simulink model "qless_forgetting_factor_16x16_nofifo"  (R2021a)
settings: Solver=FixedStepDiscrete  StartTime=0.0  StopTime=stoptime*inf  RelTol=1e-3
InitFcn:
  | qless_init_16chan_fi
undefined symbols (not defined in the file): fc, numArrayElements, physconst, srcAngles, Ts
libraries: hdlsllib x137, commfilt2 x4, commrfcorlib x3, commsync2 x3, commrflib2 x2, commrandsrc3 x2, simulink x2, phasedtxrxlib x2, commdigbbndcpm2 x1, embreciprocals x1, commdigbbndpm3 x1
(part 3 of 22)

== system qless_forgetting_factor_16x16_nofifo/MVDR_QLess_HDL/Complex Partial-Systolic Matrix Solve Using Q-less QR Decomposition with Forgetting Factor Manually Tiled n=16/Complex Partial-Systolic Q-less QR with Forgetting Factor/Complex Partial-Systolic Q-less QR with Forgetting Factor Manually tiled/Complex Partial-Systolic Q-less QR Decomposition with Forgetting Factor Section Constant pivot10 ==
  "A(i, :)^T" : Inport
  validIn : Inport  Port=2
  restart : Inport  Port=3
  Complex Partial-Systolic Q-less QR Row Rotations : Subsystem  mask(QR Complex Row Rotations){n=n, pivot=pivot}
      mask prompts: n "fixed:emblib:ColumnsInA"
      mask help: fixed:emblib:ComplexRowRotationsFullDescription
      mask DialogControl n Prompt: Number of columns in matrix A
  Data Type Conversion{,2..6} (6 alike) : DataTypeConversion  OutDataTypeStr=boolean
  Forgetting Factor : Gain  Gain=forgettingFactor  OutDataTypeStr=Inherit: Same as input
  Partial-Systolic Q-less QR with Forgetting Factor Memory Controller : Subsystem  TreatAsAtomicUnit=on  mask(Burst Q-less QR QR Memory Controller){n=n}
      mask prompts: n "fixed:emblib:ColumnsInA"
      mask help: fixed:emblib:MemoryControllerDescription
      mask DialogControl n Prompt: Number of columns in matrix A
  Same Datatype : Subsystem  TreatAsAtomicUnit=on
  Terminator : Terminator
  "R(i, :)^T" : Outport  VectorParamsAs1DForOutWhenUnconnected=off
  validR : Outport  Port=2  VectorParamsAs1DForOutWhenUnconnected=off
  yOut : Outport  Port=3  VectorParamsAs1DForOutWhenUnconnected=off
  validY : Outport  Port=4  VectorParamsAs1DForOutWhenUnconnected=off
  ready : Outport  Port=5  VectorParamsAs1DForOutWhenUnconnected=off
  wires:
  "A(i, :)^T"/1 -> Same Datatype/2(Reference), Partial-Systolic Q-less QR with Forgetting Factor Memory Controller/2(aIn)
  restart/1 -> Data Type Conversion2/1
  Complex Partial-Systolic Q-less QR Row Rotations/3(validOut) -> Data Type Conversion3/1
  Partial-Systolic Q-less QR with Forgetting Factor Memory Controller/4(validOut) -> Data Type Conversion5/1
  validIn/1 -> Data Type Conversion/1
  Partial-Systolic Q-less QR with Forgetting Factor Memory Controller/2(yOut) -> Complex Partial-Systolic Q-less QR Row Rotations/2(y)
  Same Datatype/1(DataOut) -> Partial-Systolic Q-less QR with Forgetting Factor Memory Controller/1(xIn)
  Partial-Systolic Q-less QR with Forgetting Factor Memory Controller/5(ready) -> Data Type Conversion6/1
  Complex Partial-Systolic Q-less QR Row Rotations/2(yOut) -> yOut/1
  Complex Partial-Systolic Q-less QR Row Rotations/4(ready) -> Terminator/1
  Partial-Systolic Q-less QR with Forgetting Factor Memory Controller/3(process) -> Data Type Conversion4/1
  Complex Partial-Systolic Q-less QR Row Rotations/1(xOut) -> Forgetting Factor/1
  Partial-Systolic Q-less QR with Forgetting Factor Memory Controller/1(xOut) -> Complex Partial-Systolic Q-less QR Row Rotations/1(x), "R(i, :)^T"/1
  Forgetting Factor/1 -> Same Datatype/1(Data)
  Data Type Conversion/1 -> Partial-Systolic Q-less QR with Forgetting Factor Memory Controller/3(validIn)
  Data Type Conversion2/1 -> Complex Partial-Systolic Q-less QR Row Rotations/4(restart), Partial-Systolic Q-less QR with Forgetting Factor Memory Controller/5(restart)
  Data Type Conversion3/1 -> Partial-Systolic Q-less QR with Forgetting Factor Memory Controller/4(validElim), validY/1
  Data Type Conversion5/1 -> validR/1
  Data Type Conversion6/1 -> ready/1
  Data Type Conversion4/1 -> Complex Partial-Systolic Q-less QR Row Rotations/3(validIn)

== system qless_forgetting_factor_16x16_nofifo/MVDR_QLess_HDL/Complex Partial-Systolic Matrix Solve Using Q-less QR Decomposition with Forgetting Factor Manually Tiled n=16/Complex Partial-Systolic Q-less QR with Forgetting Factor/Complex Partial-Systolic Q-less QR with Forgetting Factor Manually tiled/Complex Partial-Systolic Q-less QR Decomposition with Forgetting Factor Section Constant pivot11 ==
  "A(i, :)^T" : Inport
  validIn : Inport  Port=2
  restart : Inport  Port=3
  Complex Partial-Systolic Q-less QR Row Rotations : Subsystem  mask(QR Complex Row Rotations){n=n, pivot=pivot}
      mask prompts: n "fixed:emblib:ColumnsInA"
      mask help: fixed:emblib:ComplexRowRotationsFullDescription
      mask DialogControl n Prompt: Number of columns in matrix A
  Data Type Conversion{,2..6} (6 alike) : DataTypeConversion  OutDataTypeStr=boolean
  Forgetting Factor : Gain  Gain=forgettingFactor  OutDataTypeStr=Inherit: Same as input
  Partial-Systolic Q-less QR with Forgetting Factor Memory Controller : Subsystem  TreatAsAtomicUnit=on  mask(Burst Q-less QR QR Memory Controller){n=n}
      mask prompts: n "fixed:emblib:ColumnsInA"
      mask help: fixed:emblib:MemoryControllerDescription
      mask DialogControl n Prompt: Number of columns in matrix A
  Same Datatype : Subsystem  TreatAsAtomicUnit=on
  Terminator : Terminator
  "R(i, :)^T" : Outport  VectorParamsAs1DForOutWhenUnconnected=off
  validR : Outport  Port=2  VectorParamsAs1DForOutWhenUnconnected=off
  yOut : Outport  Port=3  VectorParamsAs1DForOutWhenUnconnected=off
  validY : Outport  Port=4  VectorParamsAs1DForOutWhenUnconnected=off
  ready : Outport  Port=5  VectorParamsAs1DForOutWhenUnconnected=off
  wires:
  "A(i, :)^T"/1 -> Same Datatype/2(Reference), Partial-Systolic Q-less QR with Forgetting Factor Memory Controller/2(aIn)
  restart/1 -> Data Type Conversion2/1
  Complex Partial-Systolic Q-less QR Row Rotations/3(validOut) -> Data Type Conversion3/1
  Partial-Systolic Q-less QR with Forgetting Factor Memory Controller/4(validOut) -> Data Type Conversion5/1
  validIn/1 -> Data Type Conversion/1
  Partial-Systolic Q-less QR with Forgetting Factor Memory Controller/2(yOut) -> Complex Partial-Systolic Q-less QR Row Rotations/2(y)
  Same Datatype/1(DataOut) -> Partial-Systolic Q-less QR with Forgetting Factor Memory Controller/1(xIn)
  Partial-Systolic Q-less QR with Forgetting Factor Memory Controller/5(ready) -> Data Type Conversion6/1
  Complex Partial-Systolic Q-less QR Row Rotations/2(yOut) -> yOut/1
  Complex Partial-Systolic Q-less QR Row Rotations/4(ready) -> Terminator/1
  Partial-Systolic Q-less QR with Forgetting Factor Memory Controller/3(process) -> Data Type Conversion4/1
  Complex Partial-Systolic Q-less QR Row Rotations/1(xOut) -> Forgetting Factor/1
  Partial-Systolic Q-less QR with Forgetting Factor Memory Controller/1(xOut) -> Complex Partial-Systolic Q-less QR Row Rotations/1(x), "R(i, :)^T"/1
  Forgetting Factor/1 -> Same Datatype/1(Data)
  Data Type Conversion/1 -> Partial-Systolic Q-less QR with Forgetting Factor Memory Controller/3(validIn)
  Data Type Conversion2/1 -> Complex Partial-Systolic Q-less QR Row Rotations/4(restart), Partial-Systolic Q-less QR with Forgetting Factor Memory Controller/5(restart)
  Data Type Conversion3/1 -> Partial-Systolic Q-less QR with Forgetting Factor Memory Controller/4(validElim), validY/1
  Data Type Conversion5/1 -> validR/1
  Data Type Conversion6/1 -> ready/1
  Data Type Conversion4/1 -> Complex Partial-Systolic Q-less QR Row Rotations/3(validIn)

== system qless_forgetting_factor_16x16_nofifo/MVDR_QLess_HDL/Complex Partial-Systolic Matrix Solve Using Q-less QR Decomposition with Forgetting Factor Manually Tiled n=16/Complex Partial-Systolic Q-less QR with Forgetting Factor/Complex Partial-Systolic Q-less QR with Forgetting Factor Manually tiled/Complex Partial-Systolic Q-less QR Decomposition with Forgetting Factor Section Constant pivot12 ==
  "A(i, :)^T" : Inport
  validIn : Inport  Port=2
  restart : Inport  Port=3
  Complex Partial-Systolic Q-less QR Row Rotations : Subsystem  mask(QR Complex Row Rotations){n=n, pivot=pivot}
      mask prompts: n "fixed:emblib:ColumnsInA"
      mask help: fixed:emblib:ComplexRowRotationsFullDescription
      mask DialogControl n Prompt: Number of columns in matrix A
  Data Type Conversion{,2..6} (6 alike) : DataTypeConversion  OutDataTypeStr=boolean
  Forgetting Factor : Gain  Gain=forgettingFactor  OutDataTypeStr=Inherit: Same as input
  Partial-Systolic Q-less QR with Forgetting Factor Memory Controller : Subsystem  TreatAsAtomicUnit=on  mask(Burst Q-less QR QR Memory Controller){n=n}
      mask prompts: n "fixed:emblib:ColumnsInA"
      mask help: fixed:emblib:MemoryControllerDescription
      mask DialogControl n Prompt: Number of columns in matrix A
  Same Datatype : Subsystem  TreatAsAtomicUnit=on
  Terminator : Terminator
  "R(i, :)^T" : Outport  VectorParamsAs1DForOutWhenUnconnected=off
  validR : Outport  Port=2  VectorParamsAs1DForOutWhenUnconnected=off
  yOut : Outport  Port=3  VectorParamsAs1DForOutWhenUnconnected=off
  validY : Outport  Port=4  VectorParamsAs1DForOutWhenUnconnected=off
  ready : Outport  Port=5  VectorParamsAs1DForOutWhenUnconnected=off
  wires:
  "A(i, :)^T"/1 -> Same Datatype/2(Reference), Partial-Systolic Q-less QR with Forgetting Factor Memory Controller/2(aIn)
  restart/1 -> Data Type Conversion2/1
  Complex Partial-Systolic Q-less QR Row Rotations/3(validOut) -> Data Type Conversion3/1
  Partial-Systolic Q-less QR with Forgetting Factor Memory Controller/4(validOut) -> Data Type Conversion5/1
  validIn/1 -> Data Type Conversion/1
  Partial-Systolic Q-less QR with Forgetting Factor Memory Controller/2(yOut) -> Complex Partial-Systolic Q-less QR Row Rotations/2(y)
  Same Datatype/1(DataOut) -> Partial-Systolic Q-less QR with Forgetting Factor Memory Controller/1(xIn)
  Partial-Systolic Q-less QR with Forgetting Factor Memory Controller/5(ready) -> Data Type Conversion6/1
  Complex Partial-Systolic Q-less QR Row Rotations/2(yOut) -> yOut/1
  Complex Partial-Systolic Q-less QR Row Rotations/4(ready) -> Terminator/1
  Partial-Systolic Q-less QR with Forgetting Factor Memory Controller/3(process) -> Data Type Conversion4/1
  Complex Partial-Systolic Q-less QR Row Rotations/1(xOut) -> Forgetting Factor/1
  Partial-Systolic Q-less QR with Forgetting Factor Memory Controller/1(xOut) -> Complex Partial-Systolic Q-less QR Row Rotations/1(x), "R(i, :)^T"/1
  Forgetting Factor/1 -> Same Datatype/1(Data)
  Data Type Conversion/1 -> Partial-Systolic Q-less QR with Forgetting Factor Memory Controller/3(validIn)
  Data Type Conversion2/1 -> Complex Partial-Systolic Q-less QR Row Rotations/4(restart), Partial-Systolic Q-less QR with Forgetting Factor Memory Controller/5(restart)
  Data Type Conversion3/1 -> Partial-Systolic Q-less QR with Forgetting Factor Memory Controller/4(validElim), validY/1
  Data Type Conversion5/1 -> validR/1
  Data Type Conversion6/1 -> ready/1
  Data Type Conversion4/1 -> Complex Partial-Systolic Q-less QR Row Rotations/3(validIn)

== system qless_forgetting_factor_16x16_nofifo/MVDR_QLess_HDL/Complex Partial-Systolic Matrix Solve Using Q-less QR Decomposition with Forgetting Factor Manually Tiled n=16/Complex Partial-Systolic Q-less QR with Forgetting Factor/Complex Partial-Systolic Q-less QR with Forgetting Factor Manually tiled/Complex Partial-Systolic Q-less QR Decomposition with Forgetting Factor Section Constant pivot13 ==
  "A(i, :)^T" : Inport
  validIn : Inport  Port=2
  restart : Inport  Port=3
  Complex Partial-Systolic Q-less QR Row Rotations : Subsystem  mask(QR Complex Row Rotations){n=n, pivot=pivot}
      mask prompts: n "fixed:emblib:ColumnsInA"
      mask help: fixed:emblib:ComplexRowRotationsFullDescription
      mask DialogControl n Prompt: Number of columns in matrix A
  Data Type Conversion{,2..6} (6 alike) : DataTypeConversion  OutDataTypeStr=boolean
  Forgetting Factor : Gain  Gain=forgettingFactor  OutDataTypeStr=Inherit: Same as input
  Partial-Systolic Q-less QR with Forgetting Factor Memory Controller : Subsystem  TreatAsAtomicUnit=on  mask(Burst Q-less QR QR Memory Controller){n=n}
      mask prompts: n "fixed:emblib:ColumnsInA"
      mask help: fixed:emblib:MemoryControllerDescription
      mask DialogControl n Prompt: Number of columns in matrix A
  Same Datatype : Subsystem  TreatAsAtomicUnit=on
  Terminator : Terminator
  "R(i, :)^T" : Outport  VectorParamsAs1DForOutWhenUnconnected=off
  validR : Outport  Port=2  VectorParamsAs1DForOutWhenUnconnected=off
  yOut : Outport  Port=3  VectorParamsAs1DForOutWhenUnconnected=off
  validY : Outport  Port=4  VectorParamsAs1DForOutWhenUnconnected=off
  ready : Outport  Port=5  VectorParamsAs1DForOutWhenUnconnected=off
  wires:
  "A(i, :)^T"/1 -> Same Datatype/2(Reference), Partial-Systolic Q-less QR with Forgetting Factor Memory Controller/2(aIn)
  restart/1 -> Data Type Conversion2/1
  Complex Partial-Systolic Q-less QR Row Rotations/3(validOut) -> Data Type Conversion3/1
  Partial-Systolic Q-less QR with Forgetting Factor Memory Controller/4(validOut) -> Data Type Conversion5/1
  validIn/1 -> Data Type Conversion/1
  Partial-Systolic Q-less QR with Forgetting Factor Memory Controller/2(yOut) -> Complex Partial-Systolic Q-less QR Row Rotations/2(y)
  Same Datatype/1(DataOut) -> Partial-Systolic Q-less QR with Forgetting Factor Memory Controller/1(xIn)
  Partial-Systolic Q-less QR with Forgetting Factor Memory Controller/5(ready) -> Data Type Conversion6/1
  Complex Partial-Systolic Q-less QR Row Rotations/2(yOut) -> yOut/1
  Complex Partial-Systolic Q-less QR Row Rotations/4(ready) -> Terminator/1
  Partial-Systolic Q-less QR with Forgetting Factor Memory Controller/3(process) -> Data Type Conversion4/1
  Complex Partial-Systolic Q-less QR Row Rotations/1(xOut) -> Forgetting Factor/1
  Partial-Systolic Q-less QR with Forgetting Factor Memory Controller/1(xOut) -> Complex Partial-Systolic Q-less QR Row Rotations/1(x), "R(i, :)^T"/1
  Forgetting Factor/1 -> Same Datatype/1(Data)
  Data Type Conversion/1 -> Partial-Systolic Q-less QR with Forgetting Factor Memory Controller/3(validIn)
  Data Type Conversion2/1 -> Complex Partial-Systolic Q-less QR Row Rotations/4(restart), Partial-Systolic Q-less QR with Forgetting Factor Memory Controller/5(restart)
  Data Type Conversion3/1 -> Partial-Systolic Q-less QR with Forgetting Factor Memory Controller/4(validElim), validY/1
  Data Type Conversion5/1 -> validR/1
  Data Type Conversion6/1 -> ready/1
  Data Type Conversion4/1 -> Complex Partial-Systolic Q-less QR Row Rotations/3(validIn)

== system qless_forgetting_factor_16x16_nofifo/MVDR_QLess_HDL/Complex Partial-Systolic Matrix Solve Using Q-less QR Decomposition with Forgetting Factor Manually Tiled n=16/Complex Partial-Systolic Q-less QR with Forgetting Factor/Complex Partial-Systolic Q-less QR with Forgetting Factor Manually tiled/Complex Partial-Systolic Q-less QR Decomposition with Forgetting Factor Section Constant pivot14 ==
  "A(i, :)^T" : Inport
  validIn : Inport  Port=2
  restart : Inport  Port=3
  Complex Partial-Systolic Q-less QR Row Rotations : Subsystem  mask(QR Complex Row Rotations){n=n, pivot=pivot}
      mask prompts: n "fixed:emblib:ColumnsInA"
      mask help: fixed:emblib:ComplexRowRotationsFullDescription
      mask DialogControl n Prompt: Number of columns in matrix A
  Data Type Conversion{,2..6} (6 alike) : DataTypeConversion  OutDataTypeStr=boolean
  Forgetting Factor : Gain  Gain=forgettingFactor  OutDataTypeStr=Inherit: Same as input
  Partial-Systolic Q-less QR with Forgetting Factor Memory Controller : Subsystem  TreatAsAtomicUnit=on  mask(Burst Q-less QR QR Memory Controller){n=n}
      mask prompts: n "fixed:emblib:ColumnsInA"
      mask help: fixed:emblib:MemoryControllerDescription
      mask DialogControl n Prompt: Number of columns in matrix A
  Same Datatype : Subsystem  TreatAsAtomicUnit=on
  Terminator : Terminator
  "R(i, :)^T" : Outport  VectorParamsAs1DForOutWhenUnconnected=off
  validR : Outport  Port=2  VectorParamsAs1DForOutWhenUnconnected=off
  yOut : Outport  Port=3  VectorParamsAs1DForOutWhenUnconnected=off
  validY : Outport  Port=4  VectorParamsAs1DForOutWhenUnconnected=off
  ready : Outport  Port=5  VectorParamsAs1DForOutWhenUnconnected=off
  wires:
  "A(i, :)^T"/1 -> Same Datatype/2(Reference), Partial-Systolic Q-less QR with Forgetting Factor Memory Controller/2(aIn)
  restart/1 -> Data Type Conversion2/1
  Complex Partial-Systolic Q-less QR Row Rotations/3(validOut) -> Data Type Conversion3/1
  Partial-Systolic Q-less QR with Forgetting Factor Memory Controller/4(validOut) -> Data Type Conversion5/1
  validIn/1 -> Data Type Conversion/1
  Partial-Systolic Q-less QR with Forgetting Factor Memory Controller/2(yOut) -> Complex Partial-Systolic Q-less QR Row Rotations/2(y)
  Same Datatype/1(DataOut) -> Partial-Systolic Q-less QR with Forgetting Factor Memory Controller/1(xIn)
  Partial-Systolic Q-less QR with Forgetting Factor Memory Controller/5(ready) -> Data Type Conversion6/1
  Complex Partial-Systolic Q-less QR Row Rotations/2(yOut) -> yOut/1
  Complex Partial-Systolic Q-less QR Row Rotations/4(ready) -> Terminator/1
  Partial-Systolic Q-less QR with Forgetting Factor Memory Controller/3(process) -> Data Type Conversion4/1
  Complex Partial-Systolic Q-less QR Row Rotations/1(xOut) -> Forgetting Factor/1
  Partial-Systolic Q-less QR with Forgetting Factor Memory Controller/1(xOut) -> Complex Partial-Systolic Q-less QR Row Rotations/1(x), "R(i, :)^T"/1
  Forgetting Factor/1 -> Same Datatype/1(Data)
  Data Type Conversion/1 -> Partial-Systolic Q-less QR with Forgetting Factor Memory Controller/3(validIn)
  Data Type Conversion2/1 -> Complex Partial-Systolic Q-less QR Row Rotations/4(restart), Partial-Systolic Q-less QR with Forgetting Factor Memory Controller/5(restart)
  Data Type Conversion3/1 -> Partial-Systolic Q-less QR with Forgetting Factor Memory Controller/4(validElim), validY/1
  Data Type Conversion5/1 -> validR/1
  Data Type Conversion6/1 -> ready/1
  Data Type Conversion4/1 -> Complex Partial-Systolic Q-less QR Row Rotations/3(validIn)

== system qless_forgetting_factor_16x16_nofifo/MVDR_QLess_HDL/Complex Partial-Systolic Matrix Solve Using Q-less QR Decomposition with Forgetting Factor Manually Tiled n=16/Complex Partial-Systolic Q-less QR with Forgetting Factor/Complex Partial-Systolic Q-less QR with Forgetting Factor Manually tiled/Complex Partial-Systolic Q-less QR Decomposition with Forgetting Factor Section Constant pivot15 ==
  "A(i, :)^T" : Inport
  validIn : Inport  Port=2
  restart : Inport  Port=3
  Complex Partial-Systolic Q-less QR Row Rotations : Subsystem  mask(QR Complex Row Rotations){n=n, pivot=pivot}
      mask prompts: n "fixed:emblib:ColumnsInA"
      mask help: fixed:emblib:ComplexRowRotationsFullDescription
      mask DialogControl n Prompt: Number of columns in matrix A
  Data Type Conversion{,2..6} (6 alike) : DataTypeConversion  OutDataTypeStr=boolean
  Forgetting Factor : Gain  Gain=forgettingFactor  OutDataTypeStr=Inherit: Same as input
  Partial-Systolic Q-less QR with Forgetting Factor Memory Controller : Subsystem  TreatAsAtomicUnit=on  mask(Burst Q-less QR QR Memory Controller){n=n}
      mask prompts: n "fixed:emblib:ColumnsInA"
      mask help: fixed:emblib:MemoryControllerDescription
      mask DialogControl n Prompt: Number of columns in matrix A
  Same Datatype : Subsystem  TreatAsAtomicUnit=on
  Terminator : Terminator
  "R(i, :)^T" : Outport  VectorParamsAs1DForOutWhenUnconnected=off
  validR : Outport  Port=2  VectorParamsAs1DForOutWhenUnconnected=off
  yOut : Outport  Port=3  VectorParamsAs1DForOutWhenUnconnected=off
  validY : Outport  Port=4  VectorParamsAs1DForOutWhenUnconnected=off
  ready : Outport  Port=5  VectorParamsAs1DForOutWhenUnconnected=off
  wires:
  "A(i, :)^T"/1 -> Same Datatype/2(Reference), Partial-Systolic Q-less QR with Forgetting Factor Memory Controller/2(aIn)
  restart/1 -> Data Type Conversion2/1
  Complex Partial-Systolic Q-less QR Row Rotations/3(validOut) -> Data Type Conversion3/1
  Partial-Systolic Q-less QR with Forgetting Factor Memory Controller/4(validOut) -> Data Type Conversion5/1
  validIn/1 -> Data Type Conversion/1
  Partial-Systolic Q-less QR with Forgetting Factor Memory Controller/2(yOut) -> Complex Partial-Systolic Q-less QR Row Rotations/2(y)
  Same Datatype/1(DataOut) -> Partial-Systolic Q-less QR with Forgetting Factor Memory Controller/1(xIn)
  Partial-Systolic Q-less QR with Forgetting Factor Memory Controller/5(ready) -> Data Type Conversion6/1
  Complex Partial-Systolic Q-less QR Row Rotations/2(yOut) -> yOut/1
  Complex Partial-Systolic Q-less QR Row Rotations/4(ready) -> Terminator/1
  Partial-Systolic Q-less QR with Forgetting Factor Memory Controller/3(process) -> Data Type Conversion4/1
  Complex Partial-Systolic Q-less QR Row Rotations/1(xOut) -> Forgetting Factor/1
  Partial-Systolic Q-less QR with Forgetting Factor Memory Controller/1(xOut) -> Complex Partial-Systolic Q-less QR Row Rotations/1(x), "R(i, :)^T"/1
  Forgetting Factor/1 -> Same Datatype/1(Data)
  Data Type Conversion/1 -> Partial-Systolic Q-less QR with Forgetting Factor Memory Controller/3(validIn)
  Data Type Conversion2/1 -> Complex Partial-Systolic Q-less QR Row Rotations/4(restart), Partial-Systolic Q-less QR with Forgetting Factor Memory Controller/5(restart)
  Data Type Conversion3/1 -> Partial-Systolic Q-less QR with Forgetting Factor Memory Controller/4(validElim), validY/1
  Data Type Conversion5/1 -> validR/1
  Data Type Conversion6/1 -> ready/1
  Data Type Conversion4/1 -> Complex Partial-Systolic Q-less QR Row Rotations/3(validIn)

== system qless_forgetting_factor_16x16_nofifo/MVDR_QLess_HDL/Complex Partial-Systolic Matrix Solve Using Q-less QR Decomposition with Forgetting Factor Manually Tiled n=16/Complex Partial-Systolic Q-less QR with Forgetting Factor/Complex Partial-Systolic Q-less QR with Forgetting Factor Manually tiled/Complex Partial-Systolic Q-less QR Decomposition with Forgetting Factor Section Constant pivot16 ==
  "A(i, :)^T" : Inport
  validIn : Inport  Port=2
  restart : Inport  Port=3
  Complex Partial-Systolic Q-less QR Row Rotations : Subsystem  mask(QR Complex Row Rotations){n=n, pivot=pivot}
      mask prompts: n "fixed:emblib:ColumnsInA"
      mask help: fixed:emblib:ComplexRowRotationsFullDescription
      mask DialogControl n Prompt: Number of columns in matrix A
  Data Type Conversion{,2..6} (6 alike) : DataTypeConversion  OutDataTypeStr=boolean
  Forgetting Factor : Gain  Gain=forgettingFactor  OutDataTypeStr=Inherit: Same as input
  Partial-Systolic Q-less QR with Forgetting Factor Memory Controller : Subsystem  TreatAsAtomicUnit=on  mask(Burst Q-less QR QR Memory Controller){n=n}
      mask prompts: n "fixed:emblib:ColumnsInA"
      mask help: fixed:emblib:MemoryControllerDescription
      mask DialogControl n Prompt: Number of columns in matrix A
  Same Datatype : Subsystem  TreatAsAtomicUnit=on
  Terminator : Terminator
  "R(i, :)^T" : Outport  VectorParamsAs1DForOutWhenUnconnected=off
  validR : Outport  Port=2  VectorParamsAs1DForOutWhenUnconnected=off
  yOut : Outport  Port=3  VectorParamsAs1DForOutWhenUnconnected=off
  validY : Outport  Port=4  VectorParamsAs1DForOutWhenUnconnected=off
  ready : Outport  Port=5  VectorParamsAs1DForOutWhenUnconnected=off
  wires:
  "A(i, :)^T"/1 -> Same Datatype/2(Reference), Partial-Systolic Q-less QR with Forgetting Factor Memory Controller/2(aIn)
  restart/1 -> Data Type Conversion2/1
  Complex Partial-Systolic Q-less QR Row Rotations/3(validOut) -> Data Type Conversion3/1
  Partial-Systolic Q-less QR with Forgetting Factor Memory Controller/4(validOut) -> Data Type Conversion5/1
  validIn/1 -> Data Type Conversion/1
  Partial-Systolic Q-less QR with Forgetting Factor Memory Controller/2(yOut) -> Complex Partial-Systolic Q-less QR Row Rotations/2(y)
  Same Datatype/1(DataOut) -> Partial-Systolic Q-less QR with Forgetting Factor Memory Controller/1(xIn)
  Partial-Systolic Q-less QR with Forgetting Factor Memory Controller/5(ready) -> Data Type Conversion6/1
  Complex Partial-Systolic Q-less QR Row Rotations/2(yOut) -> yOut/1
  Complex Partial-Systolic Q-less QR Row Rotations/4(ready) -> Terminator/1
  Partial-Systolic Q-less QR with Forgetting Factor Memory Controller/3(process) -> Data Type Conversion4/1
  Complex Partial-Systolic Q-less QR Row Rotations/1(xOut) -> Forgetting Factor/1
  Partial-Systolic Q-less QR with Forgetting Factor Memory Controller/1(xOut) -> Complex Partial-Systolic Q-less QR Row Rotations/1(x), "R(i, :)^T"/1
  Forgetting Factor/1 -> Same Datatype/1(Data)
  Data Type Conversion/1 -> Partial-Systolic Q-less QR with Forgetting Factor Memory Controller/3(validIn)
  Data Type Conversion2/1 -> Complex Partial-Systolic Q-less QR Row Rotations/4(restart), Partial-Systolic Q-less QR with Forgetting Factor Memory Controller/5(restart)
  Data Type Conversion3/1 -> Partial-Systolic Q-less QR with Forgetting Factor Memory Controller/4(validElim), validY/1
  Data Type Conversion5/1 -> validR/1
  Data Type Conversion6/1 -> ready/1
  Data Type Conversion4/1 -> Complex Partial-Systolic Q-less QR Row Rotations/3(validIn)

== system qless_forgetting_factor_16x16_nofifo/MVDR_QLess_HDL/Complex Partial-Systolic Matrix Solve Using Q-less QR Decomposition with Forgetting Factor Manually Tiled n=16/Complex Partial-Systolic Q-less QR with Forgetting Factor/Complex Partial-Systolic Q-less QR with Forgetting Factor Manually tiled/Complex Partial-Systolic Q-less QR Decomposition with Forgetting Factor Section Constant pivot2 ==
  "A(i, :)^T" : Inport
  validIn : Inport  Port=2
  restart : Inport  Port=3
  Complex Partial-Systolic Q-less QR Row Rotations : Subsystem  mask(QR Complex Row Rotations){n=n, pivot=pivot}
      mask prompts: n "fixed:emblib:ColumnsInA"
      mask help: fixed:emblib:ComplexRowRotationsFullDescription
      mask DialogControl n Prompt: Number of columns in matrix A
  Data Type Conversion{,2..6} (6 alike) : DataTypeConversion  OutDataTypeStr=boolean
  Forgetting Factor : Gain  Gain=forgettingFactor  OutDataTypeStr=Inherit: Same as input
  Partial-Systolic Q-less QR with Forgetting Factor Memory Controller : Subsystem  TreatAsAtomicUnit=on  mask(Burst Q-less QR QR Memory Controller){n=n}
      mask prompts: n "fixed:emblib:ColumnsInA"
      mask help: fixed:emblib:MemoryControllerDescription
      mask DialogControl n Prompt: Number of columns in matrix A
  Same Datatype : Subsystem  TreatAsAtomicUnit=on
  Terminator : Terminator
  "R(i, :)^T" : Outport  VectorParamsAs1DForOutWhenUnconnected=off
  validR : Outport  Port=2  VectorParamsAs1DForOutWhenUnconnected=off
  yOut : Outport  Port=3  VectorParamsAs1DForOutWhenUnconnected=off
  validY : Outport  Port=4  VectorParamsAs1DForOutWhenUnconnected=off
  ready : Outport  Port=5  VectorParamsAs1DForOutWhenUnconnected=off
  wires:
  "A(i, :)^T"/1 -> Same Datatype/2(Reference), Partial-Systolic Q-less QR with Forgetting Factor Memory Controller/2(aIn)
  restart/1 -> Data Type Conversion2/1
  Complex Partial-Systolic Q-less QR Row Rotations/3(validOut) -> Data Type Conversion3/1
  Partial-Systolic Q-less QR with Forgetting Factor Memory Controller/4(validOut) -> Data Type Conversion5/1
  validIn/1 -> Data Type Conversion/1
  Partial-Systolic Q-less QR with Forgetting Factor Memory Controller/2(yOut) -> Complex Partial-Systolic Q-less QR Row Rotations/2(y)
  Same Datatype/1(DataOut) -> Partial-Systolic Q-less QR with Forgetting Factor Memory Controller/1(xIn)
  Partial-Systolic Q-less QR with Forgetting Factor Memory Controller/5(ready) -> Data Type Conversion6/1
  Complex Partial-Systolic Q-less QR Row Rotations/2(yOut) -> yOut/1
  Complex Partial-Systolic Q-less QR Row Rotations/4(ready) -> Terminator/1
  Partial-Systolic Q-less QR with Forgetting Factor Memory Controller/3(process) -> Data Type Conversion4/1
  Complex Partial-Systolic Q-less QR Row Rotations/1(xOut) -> Forgetting Factor/1
  Partial-Systolic Q-less QR with Forgetting Factor Memory Controller/1(xOut) -> Complex Partial-Systolic Q-less QR Row Rotations/1(x), "R(i, :)^T"/1
  Forgetting Factor/1 -> Same Datatype/1(Data)
  Data Type Conversion/1 -> Partial-Systolic Q-less QR with Forgetting Factor Memory Controller/3(validIn)
  Data Type Conversion2/1 -> Complex Partial-Systolic Q-less QR Row Rotations/4(restart), Partial-Systolic Q-less QR with Forgetting Factor Memory Controller/5(restart)
  Data Type Conversion3/1 -> Partial-Systolic Q-less QR with Forgetting Factor Memory Controller/4(validElim), validY/1
  Data Type Conversion5/1 -> validR/1
  Data Type Conversion6/1 -> ready/1
  Data Type Conversion4/1 -> Complex Partial-Systolic Q-less QR Row Rotations/3(validIn)

== system qless_forgetting_factor_16x16_nofifo/MVDR_QLess_HDL/Complex Partial-Systolic Matrix Solve Using Q-less QR Decomposition with Forgetting Factor Manually Tiled n=16/Complex Partial-Systolic Q-less QR with Forgetting Factor/Complex Partial-Systolic Q-less QR with Forgetting Factor Manually tiled/Complex Partial-Systolic Q-less QR Decomposition with Forgetting Factor Section Constant pivot3 ==
  "A(i, :)^T" : Inport
  validIn : Inport  Port=2
  restart : Inport  Port=3
  Complex Partial-Systolic Q-less QR Row Rotations : Subsystem  mask(QR Complex Row Rotations){n=n, pivot=pivot}
      mask prompts: n "fixed:emblib:ColumnsInA"
      mask help: fixed:emblib:ComplexRowRotationsFullDescription
      mask DialogControl n Prompt: Number of columns in matrix A
  Data Type Conversion{,2..6} (6 alike) : DataTypeConversion  OutDataTypeStr=boolean
  Forgetting Factor : Gain  Gain=forgettingFactor  OutDataTypeStr=Inherit: Same as input
  Partial-Systolic Q-less QR with Forgetting Factor Memory Controller : Subsystem  TreatAsAtomicUnit=on  mask(Burst Q-less QR QR Memory Controller){n=n}
      mask prompts: n "fixed:emblib:ColumnsInA"
      mask help: fixed:emblib:MemoryControllerDescription
      mask DialogControl n Prompt: Number of columns in matrix A
  Same Datatype : Subsystem  TreatAsAtomicUnit=on
  Terminator : Terminator
  "R(i, :)^T" : Outport  VectorParamsAs1DForOutWhenUnconnected=off
  validR : Outport  Port=2  VectorParamsAs1DForOutWhenUnconnected=off
  yOut : Outport  Port=3  VectorParamsAs1DForOutWhenUnconnected=off
  validY : Outport  Port=4  VectorParamsAs1DForOutWhenUnconnected=off
  ready : Outport  Port=5  VectorParamsAs1DForOutWhenUnconnected=off
  wires:
  "A(i, :)^T"/1 -> Same Datatype/2(Reference), Partial-Systolic Q-less QR with Forgetting Factor Memory Controller/2(aIn)
  restart/1 -> Data Type Conversion2/1
  Complex Partial-Systolic Q-less QR Row Rotations/3(validOut) -> Data Type Conversion3/1
  Partial-Systolic Q-less QR with Forgetting Factor Memory Controller/4(validOut) -> Data Type Conversion5/1
  validIn/1 -> Data Type Conversion/1
  Partial-Systolic Q-less QR with Forgetting Factor Memory Controller/2(yOut) -> Complex Partial-Systolic Q-less QR Row Rotations/2(y)
  Same Datatype/1(DataOut) -> Partial-Systolic Q-less QR with Forgetting Factor Memory Controller/1(xIn)
  Partial-Systolic Q-less QR with Forgetting Factor Memory Controller/5(ready) -> Data Type Conversion6/1
  Complex Partial-Systolic Q-less QR Row Rotations/2(yOut) -> yOut/1
  Complex Partial-Systolic Q-less QR Row Rotations/4(ready) -> Terminator/1
  Partial-Systolic Q-less QR with Forgetting Factor Memory Controller/3(process) -> Data Type Conversion4/1
  Complex Partial-Systolic Q-less QR Row Rotations/1(xOut) -> Forgetting Factor/1
  Partial-Systolic Q-less QR with Forgetting Factor Memory Controller/1(xOut) -> Complex Partial-Systolic Q-less QR Row Rotations/1(x), "R(i, :)^T"/1
  Forgetting Factor/1 -> Same Datatype/1(Data)
  Data Type Conversion/1 -> Partial-Systolic Q-less QR with Forgetting Factor Memory Controller/3(validIn)
  Data Type Conversion2/1 -> Complex Partial-Systolic Q-less QR Row Rotations/4(restart), Partial-Systolic Q-less QR with Forgetting Factor Memory Controller/5(restart)
  Data Type Conversion3/1 -> Partial-Systolic Q-less QR with Forgetting Factor Memory Controller/4(validElim), validY/1
  Data Type Conversion5/1 -> validR/1
  Data Type Conversion6/1 -> ready/1
  Data Type Conversion4/1 -> Complex Partial-Systolic Q-less QR Row Rotations/3(validIn)

== system qless_forgetting_factor_16x16_nofifo/MVDR_QLess_HDL/Complex Partial-Systolic Matrix Solve Using Q-less QR Decomposition with Forgetting Factor Manually Tiled n=16/Complex Partial-Systolic Q-less QR with Forgetting Factor/Complex Partial-Systolic Q-less QR with Forgetting Factor Manually tiled/Complex Partial-Systolic Q-less QR Decomposition with Forgetting Factor Section Constant pivot4 ==
  "A(i, :)^T" : Inport
  validIn : Inport  Port=2
  restart : Inport  Port=3
  Complex Partial-Systolic Q-less QR Row Rotations : Subsystem  mask(QR Complex Row Rotations){n=n, pivot=pivot}
      mask prompts: n "fixed:emblib:ColumnsInA"
      mask help: fixed:emblib:ComplexRowRotationsFullDescription
      mask DialogControl n Prompt: Number of columns in matrix A
  Data Type Conversion{,2..6} (6 alike) : DataTypeConversion  OutDataTypeStr=boolean
  Forgetting Factor : Gain  Gain=forgettingFactor  OutDataTypeStr=Inherit: Same as input
  Partial-Systolic Q-less QR with Forgetting Factor Memory Controller : Subsystem  TreatAsAtomicUnit=on  mask(Burst Q-less QR QR Memory Controller){n=n}
      mask prompts: n "fixed:emblib:ColumnsInA"
      mask help: fixed:emblib:MemoryControllerDescription
      mask DialogControl n Prompt: Number of columns in matrix A
  Same Datatype : Subsystem  TreatAsAtomicUnit=on
  Terminator : Terminator
  "R(i, :)^T" : Outport  VectorParamsAs1DForOutWhenUnconnected=off
  validR : Outport  Port=2  VectorParamsAs1DForOutWhenUnconnected=off
  yOut : Outport  Port=3  VectorParamsAs1DForOutWhenUnconnected=off
  validY : Outport  Port=4  VectorParamsAs1DForOutWhenUnconnected=off
  ready : Outport  Port=5  VectorParamsAs1DForOutWhenUnconnected=off
  wires:
  "A(i, :)^T"/1 -> Same Datatype/2(Reference), Partial-Systolic Q-less QR with Forgetting Factor Memory Controller/2(aIn)
  restart/1 -> Data Type Conversion2/1
  Complex Partial-Systolic Q-less QR Row Rotations/3(validOut) -> Data Type Conversion3/1
  Partial-Systolic Q-less QR with Forgetting Factor Memory Controller/4(validOut) -> Data Type Conversion5/1
  validIn/1 -> Data Type Conversion/1
  Partial-Systolic Q-less QR with Forgetting Factor Memory Controller/2(yOut) -> Complex Partial-Systolic Q-less QR Row Rotations/2(y)
  Same Datatype/1(DataOut) -> Partial-Systolic Q-less QR with Forgetting Factor Memory Controller/1(xIn)
  Partial-Systolic Q-less QR with Forgetting Factor Memory Controller/5(ready) -> Data Type Conversion6/1
  Complex Partial-Systolic Q-less QR Row Rotations/2(yOut) -> yOut/1
  Complex Partial-Systolic Q-less QR Row Rotations/4(ready) -> Terminator/1
  Partial-Systolic Q-less QR with Forgetting Factor Memory Controller/3(process) -> Data Type Conversion4/1
  Complex Partial-Systolic Q-less QR Row Rotations/1(xOut) -> Forgetting Factor/1
  Partial-Systolic Q-less QR with Forgetting Factor Memory Controller/1(xOut) -> Complex Partial-Systolic Q-less QR Row Rotations/1(x), "R(i, :)^T"/1
  Forgetting Factor/1 -> Same Datatype/1(Data)
  Data Type Conversion/1 -> Partial-Systolic Q-less QR with Forgetting Factor Memory Controller/3(validIn)
  Data Type Conversion2/1 -> Complex Partial-Systolic Q-less QR Row Rotations/4(restart), Partial-Systolic Q-less QR with Forgetting Factor Memory Controller/5(restart)
  Data Type Conversion3/1 -> Partial-Systolic Q-less QR with Forgetting Factor Memory Controller/4(validElim), validY/1
  Data Type Conversion5/1 -> validR/1
  Data Type Conversion6/1 -> ready/1
  Data Type Conversion4/1 -> Complex Partial-Systolic Q-less QR Row Rotations/3(validIn)

== system qless_forgetting_factor_16x16_nofifo/MVDR_QLess_HDL/Complex Partial-Systolic Matrix Solve Using Q-less QR Decomposition with Forgetting Factor Manually Tiled n=16/Complex Partial-Systolic Q-less QR with Forgetting Factor/Complex Partial-Systolic Q-less QR with Forgetting Factor Manually tiled/Complex Partial-Systolic Q-less QR Decomposition with Forgetting Factor Section Constant pivot5 ==
  "A(i, :)^T" : Inport
  validIn : Inport  Port=2
  restart : Inport  Port=3
  Complex Partial-Systolic Q-less QR Row Rotations : Subsystem  mask(QR Complex Row Rotations){n=n, pivot=pivot}
      mask prompts: n "fixed:emblib:ColumnsInA"
      mask help: fixed:emblib:ComplexRowRotationsFullDescription
      mask DialogControl n Prompt: Number of columns in matrix A
  Data Type Conversion{,2..6} (6 alike) : DataTypeConversion  OutDataTypeStr=boolean
  Forgetting Factor : Gain  Gain=forgettingFactor  OutDataTypeStr=Inherit: Same as input
  Partial-Systolic Q-less QR with Forgetting Factor Memory Controller : Subsystem  TreatAsAtomicUnit=on  mask(Burst Q-less QR QR Memory Controller){n=n}
      mask prompts: n "fixed:emblib:ColumnsInA"
      mask help: fixed:emblib:MemoryControllerDescription
      mask DialogControl n Prompt: Number of columns in matrix A
  Same Datatype : Subsystem  TreatAsAtomicUnit=on
  Terminator : Terminator
  "R(i, :)^T" : Outport  VectorParamsAs1DForOutWhenUnconnected=off
  validR : Outport  Port=2  VectorParamsAs1DForOutWhenUnconnected=off
  yOut : Outport  Port=3  VectorParamsAs1DForOutWhenUnconnected=off
  validY : Outport  Port=4  VectorParamsAs1DForOutWhenUnconnected=off
  ready : Outport  Port=5  VectorParamsAs1DForOutWhenUnconnected=off
  wires:
  "A(i, :)^T"/1 -> Same Datatype/2(Reference), Partial-Systolic Q-less QR with Forgetting Factor Memory Controller/2(aIn)
  restart/1 -> Data Type Conversion2/1
  Complex Partial-Systolic Q-less QR Row Rotations/3(validOut) -> Data Type Conversion3/1
  Partial-Systolic Q-less QR with Forgetting Factor Memory Controller/4(validOut) -> Data Type Conversion5/1
  validIn/1 -> Data Type Conversion/1
  Partial-Systolic Q-less QR with Forgetting Factor Memory Controller/2(yOut) -> Complex Partial-Systolic Q-less QR Row Rotations/2(y)
  Same Datatype/1(DataOut) -> Partial-Systolic Q-less QR with Forgetting Factor Memory Controller/1(xIn)
  Partial-Systolic Q-less QR with Forgetting Factor Memory Controller/5(ready) -> Data Type Conversion6/1
  Complex Partial-Systolic Q-less QR Row Rotations/2(yOut) -> yOut/1
  Complex Partial-Systolic Q-less QR Row Rotations/4(ready) -> Terminator/1
  Partial-Systolic Q-less QR with Forgetting Factor Memory Controller/3(process) -> Data Type Conversion4/1
  Complex Partial-Systolic Q-less QR Row Rotations/1(xOut) -> Forgetting Factor/1
  Partial-Systolic Q-less QR with Forgetting Factor Memory Controller/1(xOut) -> Complex Partial-Systolic Q-less QR Row Rotations/1(x), "R(i, :)^T"/1
  Forgetting Factor/1 -> Same Datatype/1(Data)
  Data Type Conversion/1 -> Partial-Systolic Q-less QR with Forgetting Factor Memory Controller/3(validIn)
  Data Type Conversion2/1 -> Complex Partial-Systolic Q-less QR Row Rotations/4(restart), Partial-Systolic Q-less QR with Forgetting Factor Memory Controller/5(restart)
  Data Type Conversion3/1 -> Partial-Systolic Q-less QR with Forgetting Factor Memory Controller/4(validElim), validY/1
  Data Type Conversion5/1 -> validR/1
  Data Type Conversion6/1 -> ready/1
  Data Type Conversion4/1 -> Complex Partial-Systolic Q-less QR Row Rotations/3(validIn)

== system qless_forgetting_factor_16x16_nofifo/MVDR_QLess_HDL/Complex Partial-Systolic Matrix Solve Using Q-less QR Decomposition with Forgetting Factor Manually Tiled n=16/Complex Partial-Systolic Q-less QR with Forgetting Factor/Complex Partial-Systolic Q-less QR with Forgetting Factor Manually tiled/Complex Partial-Systolic Q-less QR Decomposition with Forgetting Factor Section Constant pivot6 ==
  "A(i, :)^T" : Inport
  validIn : Inport  Port=2
  restart : Inport  Port=3
  Complex Partial-Systolic Q-less QR Row Rotations : Subsystem  mask(QR Complex Row Rotations){n=n, pivot=pivot}
      mask prompts: n "fixed:emblib:ColumnsInA"
      mask help: fixed:emblib:ComplexRowRotationsFullDescription
      mask DialogControl n Prompt: Number of columns in matrix A
  Data Type Conversion{,2..6} (6 alike) : DataTypeConversion  OutDataTypeStr=boolean
  Forgetting Factor : Gain  Gain=forgettingFactor  OutDataTypeStr=Inherit: Same as input
  Partial-Systolic Q-less QR with Forgetting Factor Memory Controller : Subsystem  TreatAsAtomicUnit=on  mask(Burst Q-less QR QR Memory Controller){n=n}
      mask prompts: n "fixed:emblib:ColumnsInA"
      mask help: fixed:emblib:MemoryControllerDescription
      mask DialogControl n Prompt: Number of columns in matrix A
  Same Datatype : Subsystem  TreatAsAtomicUnit=on
  Terminator : Terminator
  "R(i, :)^T" : Outport  VectorParamsAs1DForOutWhenUnconnected=off
  validR : Outport  Port=2  VectorParamsAs1DForOutWhenUnconnected=off
  yOut : Outport  Port=3  VectorParamsAs1DForOutWhenUnconnected=off
  validY : Outport  Port=4  VectorParamsAs1DForOutWhenUnconnected=off
  ready : Outport  Port=5  VectorParamsAs1DForOutWhenUnconnected=off
  wires:
  "A(i, :)^T"/1 -> Same Datatype/2(Reference), Partial-Systolic Q-less QR with Forgetting Factor Memory Controller/2(aIn)
  restart/1 -> Data Type Conversion2/1
  Complex Partial-Systolic Q-less QR Row Rotations/3(validOut) -> Data Type Conversion3/1
  Partial-Systolic Q-less QR with Forgetting Factor Memory Controller/4(validOut) -> Data Type Conversion5/1
  validIn/1 -> Data Type Conversion/1
  Partial-Systolic Q-less QR with Forgetting Factor Memory Controller/2(yOut) -> Complex Partial-Systolic Q-less QR Row Rotations/2(y)
  Same Datatype/1(DataOut) -> Partial-Systolic Q-less QR with Forgetting Factor Memory Controller/1(xIn)
  Partial-Systolic Q-less QR with Forgetting Factor Memory Controller/5(ready) -> Data Type Conversion6/1
  Complex Partial-Systolic Q-less QR Row Rotations/2(yOut) -> yOut/1
  Complex Partial-Systolic Q-less QR Row Rotations/4(ready) -> Terminator/1
  Partial-Systolic Q-less QR with Forgetting Factor Memory Controller/3(process) -> Data Type Conversion4/1
  Complex Partial-Systolic Q-less QR Row Rotations/1(xOut) -> Forgetting Factor/1
  Partial-Systolic Q-less QR with Forgetting Factor Memory Controller/1(xOut) -> Complex Partial-Systolic Q-less QR Row Rotations/1(x), "R(i, :)^T"/1
  Forgetting Factor/1 -> Same Datatype/1(Data)
  Data Type Conversion/1 -> Partial-Systolic Q-less QR with Forgetting Factor Memory Controller/3(validIn)
  Data Type Conversion2/1 -> Complex Partial-Systolic Q-less QR Row Rotations/4(restart), Partial-Systolic Q-less QR with Forgetting Factor Memory Controller/5(restart)
  Data Type Conversion3/1 -> Partial-Systolic Q-less QR with Forgetting Factor Memory Controller/4(validElim), validY/1
  Data Type Conversion5/1 -> validR/1
  Data Type Conversion6/1 -> ready/1
  Data Type Conversion4/1 -> Complex Partial-Systolic Q-less QR Row Rotations/3(validIn)

== system qless_forgetting_factor_16x16_nofifo/MVDR_QLess_HDL/Complex Partial-Systolic Matrix Solve Using Q-less QR Decomposition with Forgetting Factor Manually Tiled n=16/Complex Partial-Systolic Q-less QR with Forgetting Factor/Complex Partial-Systolic Q-less QR with Forgetting Factor Manually tiled/Complex Partial-Systolic Q-less QR Decomposition with Forgetting Factor Section Constant pivot7 ==
  "A(i, :)^T" : Inport
  validIn : Inport  Port=2
  restart : Inport  Port=3
  Complex Partial-Systolic Q-less QR Row Rotations : Subsystem  mask(QR Complex Row Rotations){n=n, pivot=pivot}
      mask prompts: n "fixed:emblib:ColumnsInA"
      mask help: fixed:emblib:ComplexRowRotationsFullDescription
      mask DialogControl n Prompt: Number of columns in matrix A
  Data Type Conversion{,2..6} (6 alike) : DataTypeConversion  OutDataTypeStr=boolean
  Forgetting Factor : Gain  Gain=forgettingFactor  OutDataTypeStr=Inherit: Same as input
  Partial-Systolic Q-less QR with Forgetting Factor Memory Controller : Subsystem  TreatAsAtomicUnit=on  mask(Burst Q-less QR QR Memory Controller){n=n}
      mask prompts: n "fixed:emblib:ColumnsInA"
      mask help: fixed:emblib:MemoryControllerDescription
      mask DialogControl n Prompt: Number of columns in matrix A
  Same Datatype : Subsystem  TreatAsAtomicUnit=on
  Terminator : Terminator
  "R(i, :)^T" : Outport  VectorParamsAs1DForOutWhenUnconnected=off
  validR : Outport  Port=2  VectorParamsAs1DForOutWhenUnconnected=off
  yOut : Outport  Port=3  VectorParamsAs1DForOutWhenUnconnected=off
  validY : Outport  Port=4  VectorParamsAs1DForOutWhenUnconnected=off
  ready : Outport  Port=5  VectorParamsAs1DForOutWhenUnconnected=off
  wires:
  "A(i, :)^T"/1 -> Same Datatype/2(Reference), Partial-Systolic Q-less QR with Forgetting Factor Memory Controller/2(aIn)
  restart/1 -> Data Type Conversion2/1
  Complex Partial-Systolic Q-less QR Row Rotations/3(validOut) -> Data Type Conversion3/1
  Partial-Systolic Q-less QR with Forgetting Factor Memory Controller/4(validOut) -> Data Type Conversion5/1
  validIn/1 -> Data Type Conversion/1
  Partial-Systolic Q-less QR with Forgetting Factor Memory Controller/2(yOut) -> Complex Partial-Systolic Q-less QR Row Rotations/2(y)
  Same Datatype/1(DataOut) -> Partial-Systolic Q-less QR with Forgetting Factor Memory Controller/1(xIn)
  Partial-Systolic Q-less QR with Forgetting Factor Memory Controller/5(ready) -> Data Type Conversion6/1
  Complex Partial-Systolic Q-less QR Row Rotations/2(yOut) -> yOut/1
  Complex Partial-Systolic Q-less QR Row Rotations/4(ready) -> Terminator/1
  Partial-Systolic Q-less QR with Forgetting Factor Memory Controller/3(process) -> Data Type Conversion4/1
  Complex Partial-Systolic Q-less QR Row Rotations/1(xOut) -> Forgetting Factor/1
  Partial-Systolic Q-less QR with Forgetting Factor Memory Controller/1(xOut) -> Complex Partial-Systolic Q-less QR Row Rotations/1(x), "R(i, :)^T"/1
  Forgetting Factor/1 -> Same Datatype/1(Data)
  Data Type Conversion/1 -> Partial-Systolic Q-less QR with Forgetting Factor Memory Controller/3(validIn)
  Data Type Conversion2/1 -> Complex Partial-Systolic Q-less QR Row Rotations/4(restart), Partial-Systolic Q-less QR with Forgetting Factor Memory Controller/5(restart)
  Data Type Conversion3/1 -> Partial-Systolic Q-less QR with Forgetting Factor Memory Controller/4(validElim), validY/1
  Data Type Conversion5/1 -> validR/1
  Data Type Conversion6/1 -> ready/1
  Data Type Conversion4/1 -> Complex Partial-Systolic Q-less QR Row Rotations/3(validIn)
